simulink model "following_board"  (R2021a)
settings: Solver=VariableStepAuto  StartTime=0.0  StopTime=10.0  RelTol=1e-3
undefined symbols (not defined in the file or in its folder): selected_mission
settings Model: Creator=Devin Ranasinghe  LastModifiedBy=Devin Ranasinghe

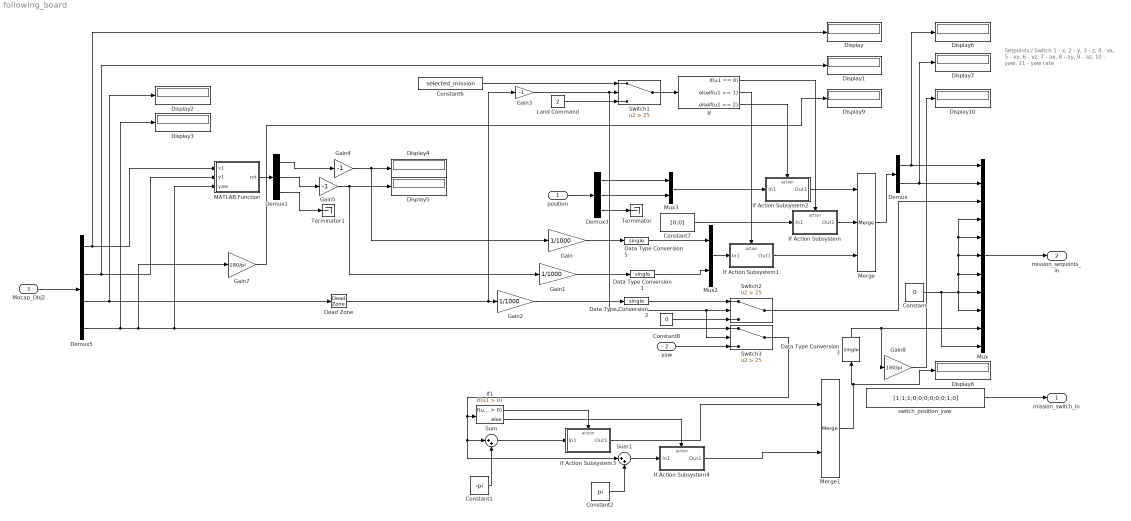
== system following_board ==
  note: Setpoints / Switch
      | 1 - x,
      | 2 - y,
      | 3 - z,
      | 4 - vx,
      | 5 - vy,
      | 6 - vz,
      | 7 - ax,
      | 8 - ay,
      | 9 - az,
      | 10 - yaw,
      | 11 - yaw rate
  position : Inport
  yaw : Inport  Port=2
  Mocap_Obj2 : Inport  Port=3
  Constant : Constant  Value=0  OutDataTypeStr=single
  Constant1 : Constant  Value=-pi
  Constant2 : Constant  Value=pi
  Constant6 : Constant  Value=selected_mission
  Constant7 : Constant  Value=[0;0]  OutDataTypeStr=single
  Constant8 : Constant  Value=0  OutDataTypeStr=single
  Data Type Conversion{1..3,5} (4 alike) : DataTypeConversion  OutDataTypeStr=single
  Dead Zone : DeadZone  LowerValue=-25  UpperValue=25  SaturateOnIntegerOverflow=on
  Demux : Demux  Outputs=2
  Demux1 : Demux  Outputs=3
  Demux3 : Demux  Outputs=3
  Demux5 : Demux
  Display{,1..10} (11 alike) : Display
  Gain : Gain  Gain=1/1000
  Gain1 : Gain  Gain=1/1000
  Gain2 : Gain  Gain=1/1000
  Gain3 : Gain  Gain=-1
  Gain4 : Gain  Gain=-1
  Gain5 : Gain  Gain=-1
  Gain7 : Gain  Gain=180/pi
  Gain8 : Gain  Gain=180/pi
  If : If  IfExpression=u1 == 0  ElseIfExpressions=u1 == 1,u1 == 2  ShowElse=off
  If Action Subsystem : Subsystem  TreatAsAtomicUnit=on
  If Action Subsystem1 : Subsystem  TreatAsAtomicUnit=on
  If Action Subsystem2 : Subsystem  TreatAsAtomicUnit=on
  If Action Subsystem3 : Subsystem  TreatAsAtomicUnit=on
  If Action Subsystem4 : Subsystem  TreatAsAtomicUnit=on
  If1 : If
  Land Command : Constant  Value=2
  MATLAB Function : MATLAB Function  TreatAsAtomicUnit=on
  Merge : Merge  Inputs=3
  Merge1 : Merge
  Mux : Mux  Inputs=11
  Mux2 : Mux  Inputs=2
  Mux3 : Mux  Inputs=2
  Sum : Sum  Inputs=|++
  Sum1 : Sum  Inputs=|++
  Switch1 : Switch  Criteria=u2 > Threshold  Threshold=25
  Switch2 : Switch  Criteria=u2 > Threshold  Threshold=25
  Switch3 : Switch  Criteria=u2 > Threshold  Threshold=25
  Terminator : Terminator
  Terminator1 : Terminator
  switch_position_yaw : Constant  Value=[1;1;1;0;0;0;0;0;0;1;0]  OutDataTypeStr=single
  mission_switch_in : Outport  VectorParamsAs1DForOutWhenUnconnected=off
  mission_setpoints_in : Outport  Port=2  VectorParamsAs1DForOutWhenUnconnected=off
  wires:
  If Action Subsystem2/1(Out1) -> Merge/1
  If1/1 -> If Action Subsystem3/Action
  switch_position_yaw/1 -> mission_switch_in/1
  Merge1/1 -> Display8/1, Data Type Conversion3/1
  Demux1/3 -> Terminator1/1
  Dead Zone/1 -> Gain3/1, Gain2/1
  Demux/1 -> Display6/1, Mux/1
  yaw/1 -> Switch3/3
  Gain3/1 -> Switch3/2, Switch2/2, Switch1/2
  Switch2/1 -> Mux/3
  Demux5/1 -> MATLAB Function/1(x1), Display/1
  Demux3/2 -> Mux3/2
  Gain2/1 -> Data Type Conversion2/1
  Mocap_Obj2/1 -> Demux5/1
  Merge/1 -> Demux/1
  If/3 -> If Action Subsystem2/Action
  Data Type Conversion1/1 -> Mux2/2
  If/1 -> If Action Subsystem/Action
  Constant6/1 -> Switch1/1
  If Action Subsystem1/1(Out1) -> Merge/3
  Demux/2 -> Display7/1, Mux/2
  Data Type Conversion3/1 -> Gain8/1, Mux/10
  Switch1/1 -> If/1
  Demux3/3 -> Terminator/1
  If Action Subsystem3/1(Out1) -> Merge1/1
  Sum/1 -> If Action Subsystem3/1(In1)
  Demux1/1 -> Gain4/1
  Demux1/2 -> Gain5/1
  Demux5/2 -> Display1/1, MATLAB Function/2(y1)
  Demux3/1 -> Mux3/1
  MATLAB Function/1(rot) -> Demux1/1
  Mux3/1 -> If Action Subsystem2/1(In1)
  Gain/1 -> Data Type Conversion5/1
  Mux/1 -> mission_setpoints_in/1
  Gain4/1 -> Gain/1, Display4/1
  position/1 -> Demux3/1
  Demux5/3 -> Dead Zone/1, Display2/1
  Sum1/1 -> If Action Subsystem4/1(In1)
  Constant2/1 -> Sum1/2
  Constant1/1 -> Sum/2
  Switch3/1 -> Sum/1, Sum1/1, If1/1
  Gain5/1 -> Gain1/1, Display5/1
  Constant/1 -> Mux/11, Mux/9, Mux/4, Mux/5, Mux/6, Mux/7, Mux/8
  Demux5/4 -> Gain7/1, Switch3/1, MATLAB Function/3(yaw), Display3/1
  Land Command/1 -> Switch1/3
  If Action Subsystem4/1(Out1) -> Merge1/2
  If Action Subsystem/1(Out1) -> Merge/2
  Data Type Conversion2/1 -> Switch2/1
  If1/2 -> If Action Subsystem4/Action
  Gain8/1 -> Display10/1
  Gain7/1 -> Display9/1
  Constant7/1 -> If Action Subsystem/1(In1)
  Mux2/1 -> If Action Subsystem1/1(In1)
  Gain1/1 -> Data Type Conversion1/1
  If/2 -> If Action Subsystem1/Action
  Data Type Conversion5/1 -> Mux2/1
  Constant8/1 -> Switch2/3

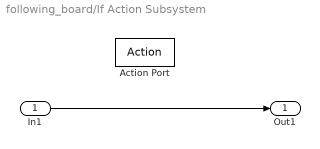
== system following_board/If Action Subsystem ==
  In1 : Inport
  Action Port : ActionPort  ActionPortLabel=if(u1 == 0)
  Out1 : Outport  VectorParamsAs1DForOutWhenUnconnected=off
  wires:
  In1/1 -> Out1/1

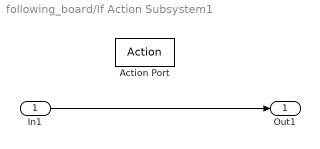
== system following_board/If Action Subsystem1 ==
  In1 : Inport
  Action Port : ActionPort  ActionPortLabel=elseif(u1 == 1)
  Out1 : Outport  VectorParamsAs1DForOutWhenUnconnected=off
  wires:
  In1/1 -> Out1/1

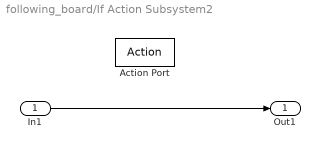
== system following_board/If Action Subsystem2 ==
  In1 : Inport
  Action Port : ActionPort  ActionPortLabel=elseif(u1 == 2)
  Out1 : Outport  VectorParamsAs1DForOutWhenUnconnected=off
  wires:
  In1/1 -> Out1/1

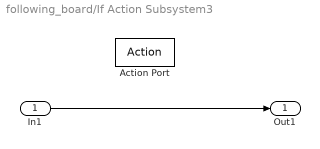
== system following_board/If Action Subsystem3 ==
  In1 : Inport
  Action Port : ActionPort  ActionPortLabel=if(u1 > 0)
  Out1 : Outport  VectorParamsAs1DForOutWhenUnconnected=off
  wires:
  In1/1 -> Out1/1

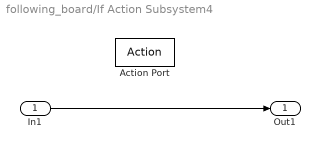
== system following_board/If Action Subsystem4 ==
  In1 : Inport
  Action Port : ActionPort  ActionPortLabel=else
  Out1 : Outport  VectorParamsAs1DForOutWhenUnconnected=off
  wires:
  In1/1 -> Out1/1

== matlab function following_board/MATLAB Function ==
  data: x1 input; rot output; y1 input; yaw input
function rot = fcn(x1,y1,yaw)
inv_rot_tra = [cos(-yaw) sin(-yaw) -x1; -sin(-yaw) cos(-yaw) -y1; 0 0 1];
rot = inv_rot_tra*[0; 30; 1];
rot(1)
